simulink model "open_loop_model"  (R2018b)
settings: Solver=VariableStepAuto  StartTime=0.0  StopTime=1  RelTol=1e-10
values from neighbouring files (symbols this model uses):
  Tl_max = 5.57    [open_loop_analysis.m]
  Vqrs_nom = 19.596    [open_loop_analysis.m]
undefined symbols (not defined in the file or in its folder): beq, Cts, Jeq, lambda_rm, Ld, Lls, Lq, Pp, r, Rs, Rts_amb, Tamb_max
settings Model: Creator=Acer  LastModifiedBy=admin

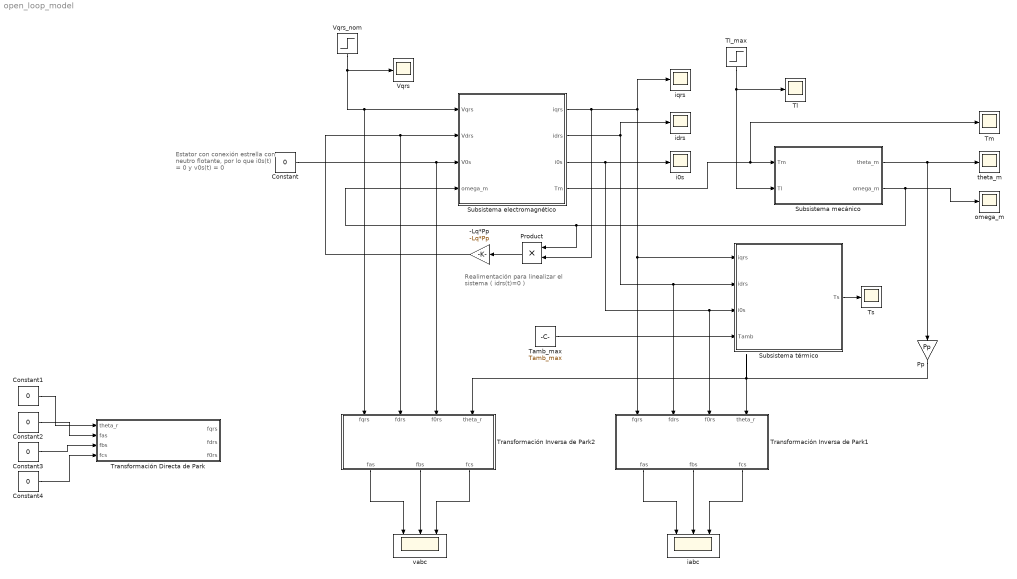
== system open_loop_model ==
  note: Estator con conexión estrella
      | con neutro flotante,
      | por lo que i0s(t) = 0 y v0s(t) = 0
  note: Realimentación para linealizar
      | el sistema ( idrs(t)=0 )
  -Lq*Pp : Gain  Gain=-Lq*Pp
  Constant{,1..4} (5 alike) : Constant  Value=0
  Pp : Gain  Gain=Pp
  Product : Product
  Subsistema electromagnético : Subsystem
  Subsistema mecánico : Subsystem
  Subsistema térmico : Subsystem
  Tamb_max : Constant  Value=Tamb_max
  Tl : Scope
  Tl_max : Step  Time=0.3  After=Tl_max  SampleTime=0
  Tm : Scope
  Transformación Directa de Park : MATLAB Function  TreatAsAtomicUnit=on
  Transformación Inversa de Park1 : MATLAB Function  TreatAsAtomicUnit=on
  Transformación Inversa de Park2 : MATLAB Function  TreatAsAtomicUnit=on
  Ts : Scope
  Vqrs : Scope
  Vqrs_nom : Step  Time=0.1  After=Vqrs_nom  SampleTime=0
  i0s : Scope
  iabc : Scope  NumInputPorts=3
  idrs : Scope
  iqrs : Scope
  omega_m : Scope
  theta_m : Scope
  vabc : Scope  NumInputPorts=3
  wires:
  Tl_max/1 -> Subsistema mecánico/2(Tl), Tl/1
  Subsistema mecánico/1(theta_m) -> theta_m/1, Pp/1
  Subsistema mecánico/2(omega_m) -> Subsistema electromagnético/4(omega_m), Product/1, omega_m/1
  Vqrs_nom/1 -> Vqrs/1, Transformación Inversa de Park2/1(fqrs), Subsistema electromagnético/1(Vqrs)
  -Lq*Pp/1 -> Transformación Inversa de Park2/2(fdrs), Subsistema electromagnético/2(Vdrs)
  Constant/1 -> Transformación Inversa de Park2/3(f0rs), Subsistema electromagnético/3(V0s)
  Subsistema electromagnético/1(iqrs) -> iqrs/1, Subsistema térmico/1(iqrs), Transformación Inversa de Park1/1(fqrs), Product/2
  Subsistema electromagnético/4(Tm) -> Subsistema mecánico/1(Tm), Tm/1
  Subsistema electromagnético/3(i0s) -> i0s/1, Subsistema térmico/3(i0s), Transformación Inversa de Park1/3(f0rs)
  Subsistema térmico/1(Ts) -> Ts/1
  Tamb_max/1 -> Subsistema térmico/4(Tamb)
  Product/1 -> -Lq*Pp/1
  Constant1/1 -> Transformación Directa de Park/1(theta_r)
  Constant2/1 -> Transformación Directa de Park/2(fas)
  Constant3/1 -> Transformación Directa de Park/3(fbs)
  Constant4/1 -> Transformación Directa de Park/4(fcs)
  Pp/1 -> Transformación Inversa de Park1/4(theta_r), Transformación Inversa de Park2/4(theta_r)
  Subsistema electromagnético/2(idrs) -> idrs/1, Subsistema térmico/2(idrs), Transformación Inversa de Park1/2(fdrs)
  Transformación Inversa de Park1/1(fas) -> iabc/1
  Transformación Inversa de Park1/3(fcs) -> iabc/3
  Transformación Inversa de Park1/2(fbs) -> iabc/2
  Transformación Inversa de Park2/1(fas) -> vabc/1
  Transformación Inversa de Park2/2(fbs) -> vabc/2
  Transformación Inversa de Park2/3(fcs) -> vabc/3

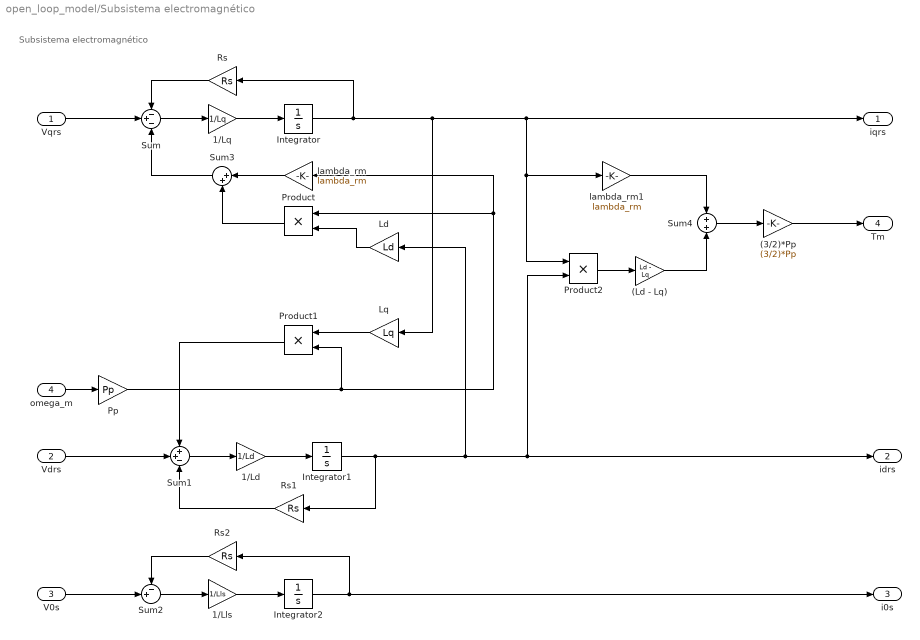
== system open_loop_model/Subsistema electromagnético ==
  note: Subsistema electromagnético
  Vqrs : Inport
  Vdrs : Inport  Port=2
  V0s : Inport  Port=3
  omega_m : Inport  Port=4
  (3/2)*Pp : Gain  Gain=(3/2)*Pp
  (Ld - Lq) : Gain  Gain=Ld - Lq
  1/Ld : Gain  Gain=1/Ld
  1/Lls : Gain  Gain=1/Lls
  1/Lq : Gain  Gain=1/Lq
  Integrator : Integrator
  Integrator1 : Integrator
  Integrator2 : Integrator
  Ld : Gain  Gain=Ld
  Lq : Gain  Gain=Lq
  Pp : Gain  Gain=Pp
  Product : Product
  Product1 : Product
  Product2 : Product
  Rs : Gain  Gain=Rs
  Rs1 : Gain  Gain=Rs
  Rs2 : Gain  Gain=Rs
  Sum : Sum  Inputs=-+-
  Sum1 : Sum  Inputs=++-
  Sum2 : Sum  Inputs=-+|
  Sum3 : Sum  Inputs=|++
  Sum4 : Sum  Inputs=+|+
  lambda_rm : Gain  Gain=lambda_rm
  lambda_rm1 : Gain  Gain=lambda_rm
  iqrs : Outport
  idrs : Outport  Port=2
  i0s : Outport  Port=3
  Tm : Outport  Port=4
  wires:
  lambda_rm/1 -> Sum3/1
  Product1/1 -> Sum1/1
  Lq/1 -> Product1/1
  Pp/1 -> lambda_rm/1, Product/1, Product1/2
  Product/1 -> Sum3/2
  Vdrs/1 -> Sum1/2
  1/Lq/1 -> Integrator/1
  Vqrs/1 -> Sum/2
  omega_m/1 -> Pp/1
  Integrator1/1 -> Ld/1, Product2/2, idrs/1, Rs1/1
  Sum1/1 -> 1/Ld/1
  Integrator/1 -> Rs/1, Lq/1, iqrs/1, Product2/1, lambda_rm1/1
  Sum2/1 -> 1/Lls/1
  Integrator2/1 -> i0s/1, Rs2/1
  Sum3/1 -> Sum/3
  Rs1/1 -> Sum1/3
  Sum4/1 -> (3/2)*Pp/1
  Ld/1 -> Product/2
  lambda_rm1/1 -> Sum4/1
  (3/2)*Pp/1 -> Tm/1
  1/Ld/1 -> Integrator1/1
  Rs2/1 -> Sum2/1
  Rs/1 -> Sum/1
  Product2/1 -> (Ld - Lq)/1
  (Ld - Lq)/1 -> Sum4/2
  Sum/1 -> 1/Lq/1
  1/Lls/1 -> Integrator2/1
  V0s/1 -> Sum2/2

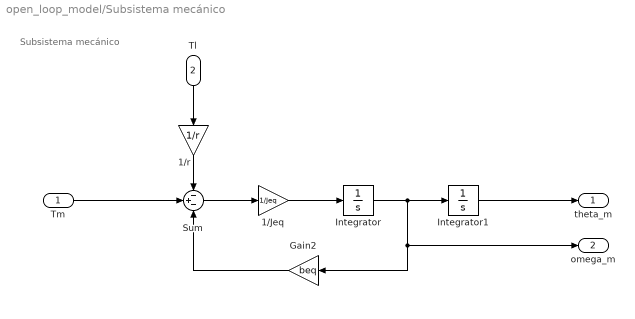
== system open_loop_model/Subsistema mecánico ==
  note: Subsistema mecánico
  Tm : Inport
  Tl : Inport  Port=2
  1/Jeq : Gain  Gain=1/Jeq
  1/r : Gain  Gain=1/r
  Gain2 : Gain  Gain=beq
  Integrator : Integrator
  Integrator1 : Integrator
  Sum : Sum  Inputs=-+-
  theta_m : Outport
  omega_m : Outport  Port=2
  wires:
  Integrator1/1 -> theta_m/1
  Integrator/1 -> omega_m/1, Gain2/1, Integrator1/1
  Tm/1 -> Sum/2
  1/r/1 -> Sum/1
  Sum/1 -> 1/Jeq/1
  Tl/1 -> 1/r/1
  Gain2/1 -> Sum/3
  1/Jeq/1 -> Integrator/1

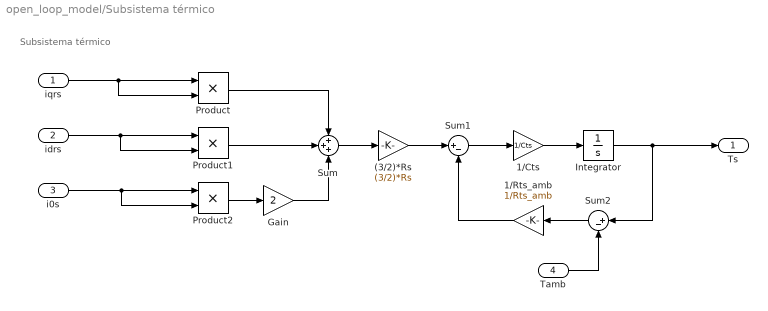
== system open_loop_model/Subsistema térmico ==
  note: Subsistema térmico
  iqrs : Inport
  idrs : Inport  Port=2
  i0s : Inport  Port=3
  Tamb : Inport  Port=4
  (3/2)*Rs : Gain  Gain=(3/2)*Rs
  1/Cts : Gain  Gain=1/Cts
  1/Rts_amb : Gain  Gain=1/Rts_amb
  Gain : Gain  Gain=2
  Integrator : Integrator  InitialCondition=Tamb_max
  Product : Product
  Product1 : Product
  Product2 : Product
  Sum : Sum  Inputs=+++
  Sum1 : Sum  Inputs=|+-
  Sum2 : Sum  Inputs=|+-
  Ts : Outport
  wires:
  Integrator/1 -> Ts/1, Sum2/1
  1/Cts/1 -> Integrator/1
  i0s/1 -> Product2/2, Product2/1
  Product/1 -> Sum/1
  Sum2/1 -> 1/Rts_amb/1
  (3/2)*Rs/1 -> Sum1/1
  Tamb/1 -> Sum2/2
  Sum/1 -> (3/2)*Rs/1
  1/Rts_amb/1 -> Sum1/2
  Gain/1 -> Sum/3
  Sum1/1 -> 1/Cts/1
  iqrs/1 -> Product/2, Product/1
  idrs/1 -> Product1/2, Product1/1
  Product2/1 -> Gain/1
  Product1/1 -> Sum/2

== matlab function open_loop_model/Transformación Inversa de Park2 ==
  data: fqrs input; fdrs input; f0rs input; theta_r input; fas output; fbs output; fcs output
function [fas, fbs, fcs] = dq0_transformation_inverse( fqrs, fdrs, f0rs, theta_r )
% TRANSFORMACIÓN INVERSA DE PARK
%   Transformación directa para pasar desde coordenadas trifásicas del
%   estator abc a las coordenadas fijas al rotor qd0.
fqd0 = [ fqrs; fdrs; f0rs ];

A = [ 
    cos(theta_r)            sin(theta_r)            1;
    cos(theta_r - 2*pi/3)   sin(theta_r - 2*pi/3)   1;
    cos(theta_r + 2*pi/3)   sin(theta_r + 2*pi/3)   1
    ];

fabc =  A * fqd0;

fas = fabc(1);
fbs = fabc(2);
fcs = fabc(3);

end

== matlab function open_loop_model/Transformación Directa de Park ==
  data: theta_r input; fas input; fqrs output; fbs input; fdrs output; fcs input; f0rs output
function [fqrs, fdrs, f0rs] = dq0_transformation_direct( theta_r, fas, fbs, fcs )
% TRANSFORMACIÓN DIRECTA DE PARK
%   Transformación directa para pasar desde coordenadas trifásicas del
%   estator abc a las coordenadas fijas al rotor qd0.
fabc = [ fas; fbs; fcs ];

A = [ 
    cos(theta_r)    cos(theta_r - 2*pi/3)   cos(theta_r + 2*pi/3);
    sin(theta_r)    sin(theta_r - 2*pi/3)   sin(theta_r + 2*pi/3);
    0.5             0.5                     0.5
    ];

fqd0 = (2/3) * A * fabc;

fqrs = fqd0(1);
fdrs = fqd0(2);
f0rs = fqd0(3);

end

== matlab function open_loop_model/Transformación Inversa de Park1 ==
  data: fqrs input; fdrs input; f0rs input; theta_r input; fas output; fbs output; fcs output
function [fas, fbs, fcs] = dq0_transformation_inverse( fqrs, fdrs, f0rs, theta_r )
% TRANSFORMACIÓN INVERSA DE PARK
%   Transformación directa para pasar desde coordenadas trifásicas del
%   estator abc a las coordenadas fijas al rotor qd0.
fqd0 = [ fqrs; fdrs; f0rs ];

A = [ 
    cos(theta_r)            sin(theta_r)            1;
    cos(theta_r - 2*pi/3)   sin(theta_r - 2*pi/3)   1;
    cos(theta_r + 2*pi/3)   sin(theta_r + 2*pi/3)   1
    ];

fabc =  A * fqd0;

fas = fabc(1);
fbs = fabc(2);
fcs = fabc(3);

end
